simulink model "ur5_simulink_ros2_pbvs_all_methods_2023b"  (R2023b)
settings: Solver=ode4  StartTime=0.0  StopTime=inf  FixedStep=0.005  RelTol=1e-3
InitFcn:
  | l=5;
model workspace (MAT data in the model file):
  SL_ROS_VariableLengthArrays_MaxSizes.CommonInfo.ArrayTruncateAction = 'EmitWarning'
  SL_ROS_VariableLengthArrays_MaxSizes.MsgTypeMap = containers.Map
  SL_ROS_VariableLengthArrays_MaxSizes.MsgTypeMap.serialization.keys = {'example_interfaces/Float64MultiArray'}
  SL_ROS_VariableLengthArrays_MaxSizes.MsgTypeMap.serialization.values{1}.PropertyName = 'data'
  SL_ROS_VariableLengthArrays_MaxSizes.MsgTypeMap.serialization.values{1}.DataType = 'double'
  SL_ROS_VariableLengthArrays_MaxSizes.MsgTypeMap.serialization.values{1}.MaxLength = 1
  SL_ROS_VariableLengthArrays_MaxSizes.MsgTypeMap.serialization.uniformity = 0
  SL_ROS_VariableLengthArrays_MaxSizes.MsgTypeMap.serialization.keyType = 'char'
  SL_ROS_VariableLengthArrays_MaxSizes.MsgTypeMap.serialization.valueType = 'any'
values from neighbouring files (symbols this model uses):
  D = zeros(6,12)    [ibvs_cstate.m]
undefined symbols (not defined in the file or in its folder): data, data_SL_Info, DiscIntNeverNeededParam
libraries: simulink x9, ros2lib x8, slpidlib x6, robotmaniplib x3, mpclib x3, robotcorelib x1
(part 1 of 2)
settings Model: SimulationMode=accelerator  Creator=81232  LastModifiedBy=Administrator
settings OptimizationCC: EnhancedBackFolding=on  PassReuseOutputArgsAs=Individual arguments  ZeroExternalMemoryAtStartup=off  ZeroInternalMemoryAtStartup=off  MaxStackSize=64  OptimizeBlockOrder=speed  DifferentSizesBufferReuse=on  OptimizationCustomize=off  EfficientTunableParamExpr=on
settings DebuggingCC: ParameterTunabilityLossMsg=error
settings ModelReferenceCC: EnableRefExpFcnMdlSchedulingChecks=on
settings SFSimCC: MATLABDynamicMemAlloc=off
settings RTWCC: Description=Embedded Coder  SystemTargetFile=ert.tlc  HardwareBoard=Robot Operating System 2 (ROS 2)  TLCOptions="-aInlineSetEventsForThisBaseRateFcn=TLC_FALSE -aSuppressMultiTaskScheduler=TLC_FALSE  -aRateBasedStepFcn=0"  TemplateMakefile=ert_default_tmf  Toolchain=Colcon Tools  TargetLang=C++
settings CodeAppCC: ForceParamTrailComments=on  IgnoreCustomStorageClasses=off  OperatorAnnotations=on  SimulinkDataObjDesc=on  SFDataObjDesc=on  InsertBlockDesc=on
settings ERTTargetCC: CodeInterfacePackaging=C++ class  RootIOFormat=Structure reference

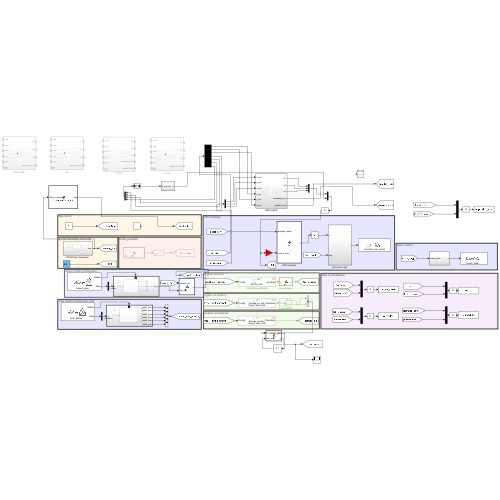
[thumbnail: Simulink's stored preview of the top-level diagram]
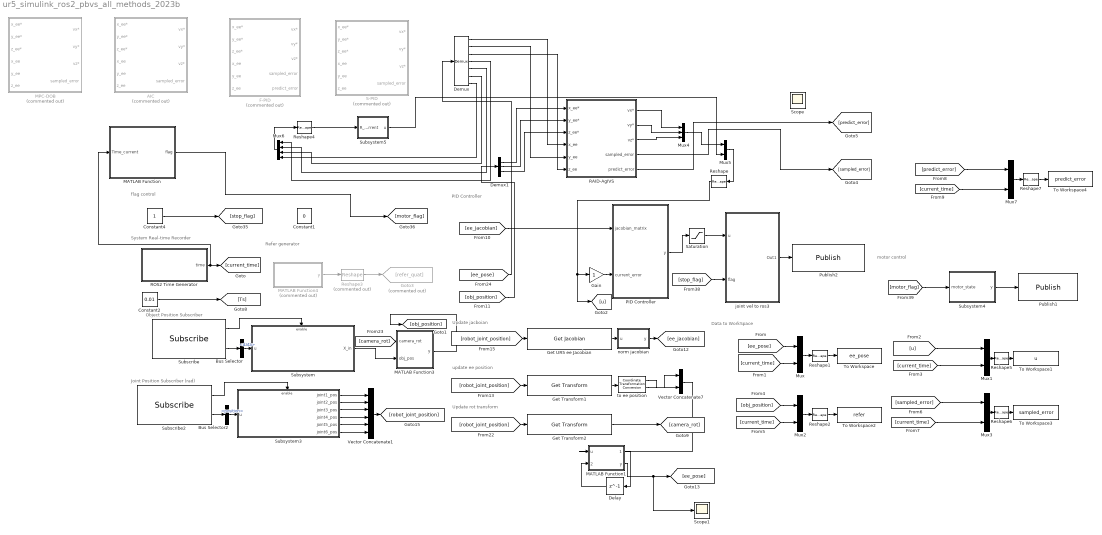
== system ur5_simulink_ros2_pbvs_all_methods_2023b ==
  note: PID Controller
  note: update ee position
  note: Joint Position Subscriber (rad)
  note: Refer generator
  note: Data to WorkSpace
  note: System Real-time Recorder
  note: Object Position Subscriber
  note: Update jacboian
  note: Update rot transform
  note: flag control
  note: motor control
  AIC : Subsystem  Commented=on
  Bus Selector : BusSelector  OutputSignals=data
  Bus Selector2 : BusSelector  OutputSignals=position
  Constant1 : Constant  Value=0
  Constant2 : Constant  Value=0.01
  Constant4 : Constant
  Delay : Delay  DelayLength=1  InitialCondition=[0;0;0;0]
  Demux : Demux  Outputs=7
  Demux1 : Demux  Outputs=3
  F-PID : Subsystem  Commented=on
  Gain : Gain
  Get Transform1 : robotmaniplib/Get Transform  RigidBodyTree=ur5_model  SourceBody=ee_link  TargetBody=base_link  SimulateUsing=Interpreted execution
  Get Transform2 : robotmaniplib/Get Transform  RigidBodyTree=ur5_model  SourceBody=camera  TargetBody=base_link  SimulateUsing=Interpreted execution
  Get UR5 ee Jacobian : robotmaniplib/Get Jacobian  RigidBodyTree=ur5_model  EndEffector=ee_link  SimulateUsing=Interpreted execution
  Goto3 : Goto  Commented=on  GotoTag=refer_quat
  MATLAB Function : MATLAB Function  TreatAsAtomicUnit=on
  MATLAB Function1 : MATLAB Function  TreatAsAtomicUnit=on
  MATLAB Function3 : MATLAB Function  TreatAsAtomicUnit=on
  MATLAB Function4 : MATLAB Function  Commented=on  TreatAsAtomicUnit=on
  MPC-DOB : Subsystem  Commented=on
  Mux{,1..3,5,7} (6 alike) : Mux  Inputs=2
  Mux4 : Mux  Inputs=3
  Mux6 : Mux
  PID Controller : MATLAB Function  TreatAsAtomicUnit=on
  Publish1 : ros2lib/Publish  topicSource=Select from ROS network  topic=/motor_state  messageType=std_msgs/Int64  QOSHistory=Keep last  QOSDepth=1  QOSReliability=Reliable  QOSDurability=Volatile
      settings: LibrarySourceBlock=roslib/ROS 2/Publish
  Publish2 : ros2lib/Publish  topicSource=Select from ROS network  topic=/simulink_mpc_result  messageType=std_msgs/Float64MultiArray  QOSHistory=Keep last  QOSDepth=1  QOSReliability=Reliable  QOSDurability=Volatile
      settings: LibrarySourceBlock=roslib/ROS 2/Publish
  RAID-AgIVS : Subsystem
  ROS2 Time Generator : Subsystem
  Reshape : Reshape  OutputDimensionality=Customize  OutputDimensions=[6,1]
  Reshape1 : Reshape  OutputDimensionality=Customize  OutputDimensions=[8]
  Reshape2 : Reshape  OutputDimensionality=Customize  OutputDimensions=[4]
  Reshape3 : Reshape  Commented=on  OutputDimensions=[1,7]
  Reshape4 : Reshape  OutputDimensionality=Row vector (2-D)
  Reshape5 : Reshape  OutputDimensionality=Customize  OutputDimensions=[7]
  Reshape6 : Reshape  OutputDimensionality=Customize  OutputDimensions=[4]
  Reshape7 : Reshape  OutputDimensionality=Customize  OutputDimensions=[4]
  S-PID : Subsystem  Commented=on
  Saturation : Saturate  UpperLimit=0.7  LowerLimit=-0.7  LinearizeAsGain=off
  Scope : Scope
  Scope1 : Scope
  Subscribe : ros2lib/Subscribe  topicSource=Select from ROS network  topic=/object_pose  messageType=std_msgs/Float64MultiArray  sampleTime=-1  QOSHistory=Keep last  QOSDepth=1  QOSReliability=Reliable  QOSDurability=Volatile
  Subscribe2 : ros2lib/Subscribe  topicSource=Select from ROS network  topic=/joint_states  messageType=sensor_msgs/JointState  sampleTime=-1  QOSHistory=Keep last  QOSDepth=1  QOSReliability=Reliable  QOSDurability=Volatile
  Subsystem : Subsystem
  Subsystem3 : Subsystem
  Subsystem4 : Subsystem
  Subsystem5 : Subsystem
  To Workspace : ToWorkspace  VariableName=ee_pose  SaveFormat=Timeseries  SampleTime=-1
  To Workspace1 : ToWorkspace  VariableName=u  SaveFormat=Timeseries  SampleTime=-1
  To Workspace2 : ToWorkspace  VariableName=refer  SaveFormat=Timeseries  SampleTime=-1
  To Workspace3 : ToWorkspace  VariableName=sampled_error  SaveFormat=Timeseries  SampleTime=-1
  To Workspace4 : ToWorkspace  VariableName=predict_error  SaveFormat=Timeseries  SampleTime=-1
  Vector Concatenate1 : Concatenate  NumInputs=6
  Vector Concatenate7 : Concatenate
  joint vel to ros3 : Subsystem
  norm jacobian : MATLAB Function  TreatAsAtomicUnit=on
  to ee position : robotcorelib/Coordinate Transformation Conversion  InputRepresentation=Homogeneous Transformation  InputEulerSequence=ZYX  ShowTrVecInputPort=on  OutputRepresentation=Quaternion  OutputEulerSequence=ZYX  ShowTrVecOutputPort=on  SimulateUsing=Interpreted execution
  wires:
  Bus Selector/1 -> Subsystem/1(u)  "<data>"
  Subscribe/2 -> Bus Selector/1
  Subscribe/1 -> Subsystem/Enable
  ROS2 Time Generator/1(time) -> [current_time], MATLAB Function/1(Time_current)
  [ee_pose] -> Mux/1
  [current_time] -> Mux/2
  [current_time] -> Mux1/2
  [current_time] -> Mux2/2
  Mux2/1 -> Reshape2/1
  [current_time] -> Mux3/2
  Mux3/1 -> Reshape6/1
  [sampled_error] -> Mux3/1
  [u] -> Mux1/1
  Mux1/1 -> Reshape5/1
  Reshape5/1 -> To Workspace1/1
  Reshape6/1 -> To Workspace3/1
  Subscribe2/2 -> Bus Selector2/1
  Bus Selector2/1 -> Subsystem3/1(u)  "<position>"
  Subscribe2/1 -> Subsystem3/Enable
  Subsystem3/1(joint1_pos) -> Vector Concatenate1/1
  Subsystem3/2(joint2_pos) -> Vector Concatenate1/2
  Subsystem3/3(joint3_pos) -> Vector Concatenate1/3
  Subsystem3/4(joint4_pos) -> Vector Concatenate1/4
  Subsystem3/5(joint5_pos) -> Vector Concatenate1/5
  Subsystem3/6(joint6_pos) -> Vector Concatenate1/6
  norm jacobian/1(y) -> [ee_jacobian]
  Get UR5 ee Jacobian/1 -> norm jacobian/1(u)
  [robot_joint_position] -> Get UR5 ee Jacobian/1
  [robot_joint_position] -> Get Transform1/1
  Vector Concatenate1/1 -> [robot_joint_position]
  Mux/1 -> Reshape1/1
  Reshape1/1 -> To Workspace/1
  Reshape2/1 -> To Workspace2/1
  [obj_position] -> Mux2/1
  Constant2/1 -> [Ts]
  Get Transform2/1 -> [camera_rot]
  MATLAB Function3/1(y) -> [obj_position]
  [camera_rot] -> MATLAB Function3/1(camera_rot)
  Subsystem/1(X_in) -> MATLAB Function3/2(obj_pos)
  Reshape3/1 -> Goto3/1
  MATLAB Function4/1(y) -> Reshape3/1
  Get Transform1/1 -> to ee position/1
  to ee position/1 -> Vector Concatenate7/2
  to ee position/2 -> Vector Concatenate7/1
  [ee_jacobian] -> PID Controller/1(jacobian_matrix)
  Saturation/1 -> joint vel to ros3/1(u)
  joint vel to ros3/1(Out1) -> Publish2/1
  PID Controller/1(y) -> Saturation/1
  Constant4/1 -> [stop_flag]
  [stop_flag] -> joint vel to ros3/2(flag)
  Mux5/1 -> Reshape/1
  Gain/1 -> PID Controller/2(current_error)
  Subsystem4/1(y) -> Publish1/1
  [motor_flag] -> Subsystem4/1(motor_state)
  [robot_joint_position] -> Get Transform2/1
  Demux/1 -> RAID-AgIVS/4(x_ee)
  Demux/2 -> RAID-AgIVS/5(y_ee)
  Demux/3 -> RAID-AgIVS/6(z_ee)
  Demux1/1 -> RAID-AgIVS/1(x_ee*)
  Demux1/2 -> RAID-AgIVS/2(y_ee*)
  Demux1/3 -> RAID-AgIVS/3(z_ee*)
  Mux4/1 -> Mux5/1
  Reshape/1 -> [u], Gain/1
  [ee_pose] -> Demux/1
  [obj_position] -> Demux1/1
  RAID-AgIVS/1(vx*) -> Mux4/1
  Demux/4 -> Mux6/1
  Demux/5 -> Mux6/2
  Demux/6 -> Mux6/3
  Demux/7 -> Mux6/4
  Mux6/1 -> Reshape4/1
  Subsystem5/1(u) -> Mux5/2
  Reshape4/1 -> Subsystem5/1(R_current)
  [current_time] -> Mux7/2
  [predict_error] -> Mux7/1
  Mux7/1 -> Reshape7/1
  Reshape7/1 -> To Workspace4/1
  Vector Concatenate7/1 -> MATLAB Function1/1(u)
  MATLAB Function1/1(current_quat) -> Delay/1
  Delay/1 -> MATLAB Function1/2(last_quat)
  MATLAB Function1/2(y) -> Scope1/1, [ee_pose]
  RAID-AgIVS/2(vy*) -> Mux4/2
  MATLAB Function/1(flag) -> [motor_flag]
  RAID-AgIVS/5(predict_error) -> [predict_error]
  RAID-AgIVS/3(vz*) -> Mux4/3
  RAID-AgIVS/4(sampled_error) -> [sampled_error]

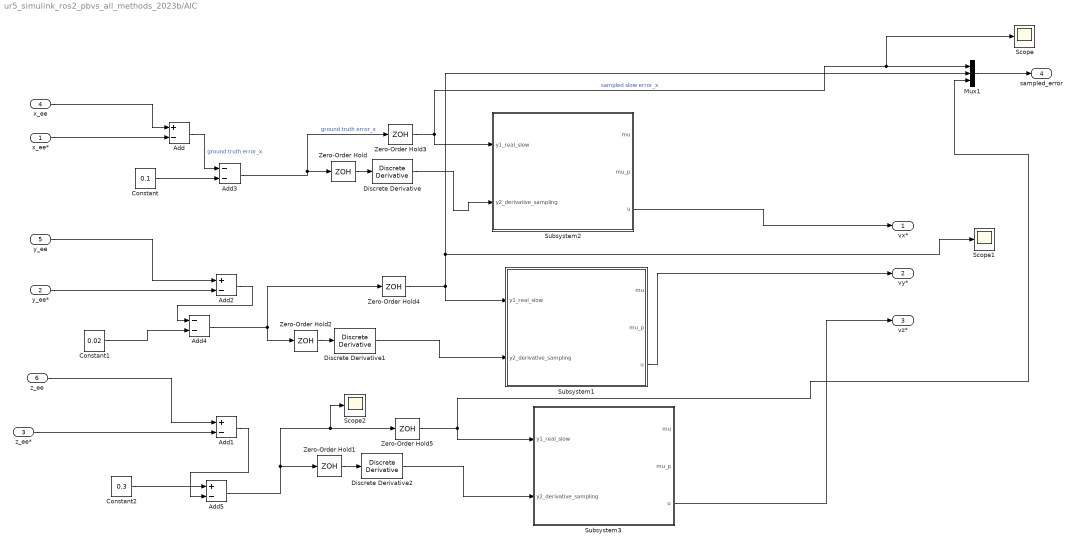
== system ur5_simulink_ros2_pbvs_all_methods_2023b/AIC ==
  x_ee* : Inport
  y_ee* : Inport  Port=2
  z_ee* : Inport  Port=3
  x_ee : Inport  Port=4
  y_ee : Inport  Port=5
  z_ee : Inport  Port=6
  Add{,1..2,5} (4 alike) : Sum  Inputs=+-
  Add3 : Sum  Inputs=--
  Add4 : Sum  Inputs=--
  Constant : Constant  Value=0.1
  Constant1 : Constant  Value=0.02
  Constant2 : Constant  Value=0.3
  Discrete Derivative : simulink/Discrete/Discrete Derivative  gainval=1.0  ICPrevScaledInput=0  OutMin=[]  OutMax=[]  OutDataType=fixdt(1, 16)  OutScaling=2^-10  DoSatur=off
  Discrete Derivative1 : simulink/Discrete/Discrete Derivative  gainval=1.0  ICPrevScaledInput=0.0  OutMin=[]  OutMax=[]  OutDataType=fixdt(1, 16)  OutScaling=2^-10  DoSatur=off
  Discrete Derivative2 : simulink/Discrete/Discrete Derivative  gainval=1.0  ICPrevScaledInput=0.0  OutMin=[]  OutMax=[]  OutDataType=fixdt(1, 16)  OutScaling=2^-10  DoSatur=off
  Mux1 : Mux  Inputs=3
  Scope : Scope
  Scope1 : Scope
  Scope2 : Scope
  Subsystem1 : Subsystem
  Subsystem2 : Subsystem
  Subsystem3 : Subsystem
  Zero-Order Hold{,1..5} (6 alike) : ZeroOrderHold  SampleTime=0.05
  vx* : Outport
  vy* : Outport  Port=2
  vz* : Outport  Port=3
  sampled_error : Outport  Port=4
  wires:
  Subsystem3/3(u) -> vz*/1
  Subsystem1/3(u) -> vy*/1
  Subsystem2/3(u) -> vx*/1
  Discrete Derivative1/1 -> Subsystem1/2(y2_derivative_sampling)
  Add1/1 -> Add5/2
  Constant/1 -> Add3/2
  Add/1 -> Add3/1  "ground truth error_x"
  z_ee*/1 -> Add1/2
  Discrete Derivative/1 -> Subsystem2/2(y2_derivative_sampling)
  y_ee*/1 -> Add2/2
  Constant2/1 -> Add5/1
  Zero-Order Hold5/1 -> Subsystem3/1(y1_real_slow), Mux1/3
  Add4/1 -> Zero-Order Hold4/1, Zero-Order Hold2/1
  x_ee*/1 -> Add/2
  x_ee/1 -> Add/1
  Zero-Order Hold1/1 -> Discrete Derivative2/1
  Zero-Order Hold/1 -> Discrete Derivative/1
  Add5/1 -> Zero-Order Hold5/1, Scope2/1, Zero-Order Hold1/1
  Zero-Order Hold3/1 -> Scope/1, Mux1/1, Subsystem2/1(y1_real_slow)  "sampled slow error_x"
  Zero-Order Hold2/1 -> Discrete Derivative1/1
  y_ee/1 -> Add2/1
  Add2/1 -> Add4/1
  Constant1/1 -> Add4/2
  Zero-Order Hold4/1 -> Subsystem1/1(y1_real_slow), Scope1/1, Mux1/2
  z_ee/1 -> Add1/1
  Add3/1 -> Zero-Order Hold3/1, Zero-Order Hold/1  "ground truth error_x"
  Discrete Derivative2/1 -> Subsystem3/2(y2_derivative_sampling)
  Mux1/1 -> sampled_error/1

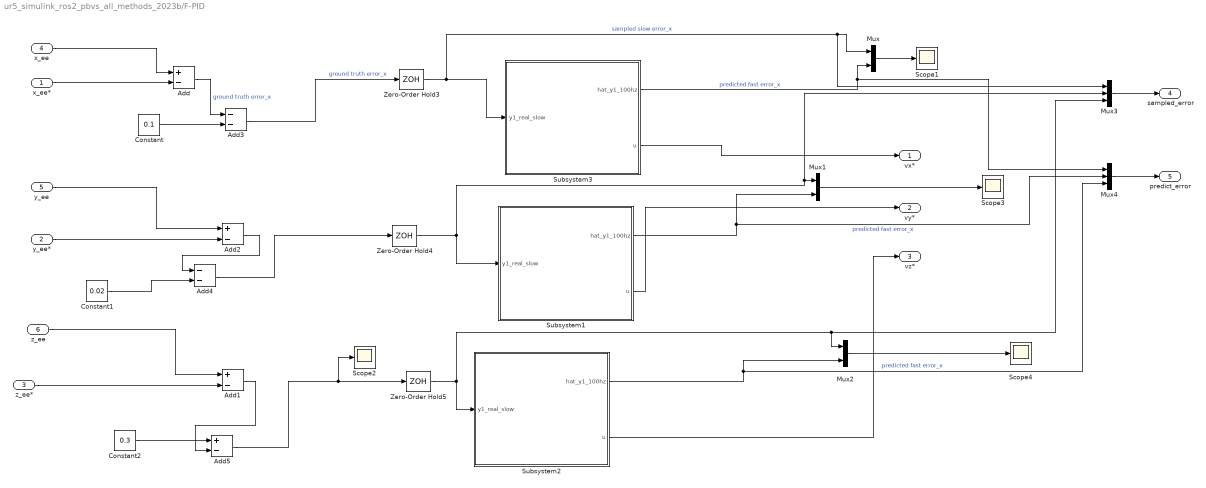
== system ur5_simulink_ros2_pbvs_all_methods_2023b/F-PID ==
  x_ee* : Inport
  y_ee* : Inport  Port=2
  z_ee* : Inport  Port=3
  x_ee : Inport  Port=4
  y_ee : Inport  Port=5
  z_ee : Inport  Port=6
  Add{,1..2,5} (4 alike) : Sum  Inputs=+-
  Add3 : Sum  Inputs=--
  Add4 : Sum  Inputs=--
  Constant : Constant  Value=0.1
  Constant1 : Constant  Value=0.02
  Constant2 : Constant  Value=0.3
  Mux : Mux  Inputs=2
  Mux1 : Mux  Inputs=2
  Mux2 : Mux  Inputs=2
  Mux3 : Mux  Inputs=3
  Mux4 : Mux  Inputs=3
  Scope{1..4} (4 alike) : Scope
  Subsystem1 : Subsystem
  Subsystem2 : Subsystem
  Subsystem3 : Subsystem
  Zero-Order Hold3 : ZeroOrderHold  SampleTime=0.05
  Zero-Order Hold4 : ZeroOrderHold  SampleTime=0.05
  Zero-Order Hold5 : ZeroOrderHold  SampleTime=0.05
  vx* : Outport
  vy* : Outport  Port=2
  vz* : Outport  Port=3
  sampled_error : Outport  Port=4
  predict_error : Outport  Port=5
  wires:
  Add4/1 -> Zero-Order Hold4/1
  x_ee/1 -> Add/1
  Add5/1 -> Zero-Order Hold5/1, Scope2/1
  Subsystem3/2(u) -> vx*/1
  Add3/1 -> Zero-Order Hold3/1  "ground truth error_x"
  x_ee*/1 -> Add/2
  y_ee/1 -> Add2/1
  z_ee/1 -> Add1/1
  Subsystem2/2(u) -> vz*/1
  y_ee*/1 -> Add2/2
  z_ee*/1 -> Add1/2
  Zero-Order Hold3/1 -> Mux3/1, Mux/1, Subsystem3/1(y1_real_slow)  "sampled slow error_x"
  Zero-Order Hold4/1 -> Subsystem1/1(y1_real_slow), Mux3/2, Mux1/1
  Subsystem1/2(u) -> vy*/1
  Subsystem3/1(hat_y1_100hz) -> Mux4/1, Mux/2  "predicted fast error_x"
  Mux/1 -> Scope1/1
  Add/1 -> Add3/1  "ground truth error_x"
  Constant/1 -> Add3/2
  Constant1/1 -> Add4/2
  Add2/1 -> Add4/1
  Constant2/1 -> Add5/1
  Add1/1 -> Add5/2
  Subsystem1/1(hat_y1_100hz) -> Mux4/2, Mux1/2  "predicted fast error_x"
  Mux1/1 -> Scope3/1
  Mux2/1 -> Scope4/1
  Zero-Order Hold5/1 -> Subsystem2/1(y1_real_slow), Mux3/3, Mux2/1
  Subsystem2/1(hat_y1_100hz) -> Mux4/3, Mux2/2  "predicted fast error_x"
  Mux3/1 -> sampled_error/1
  Mux4/1 -> predict_error/1

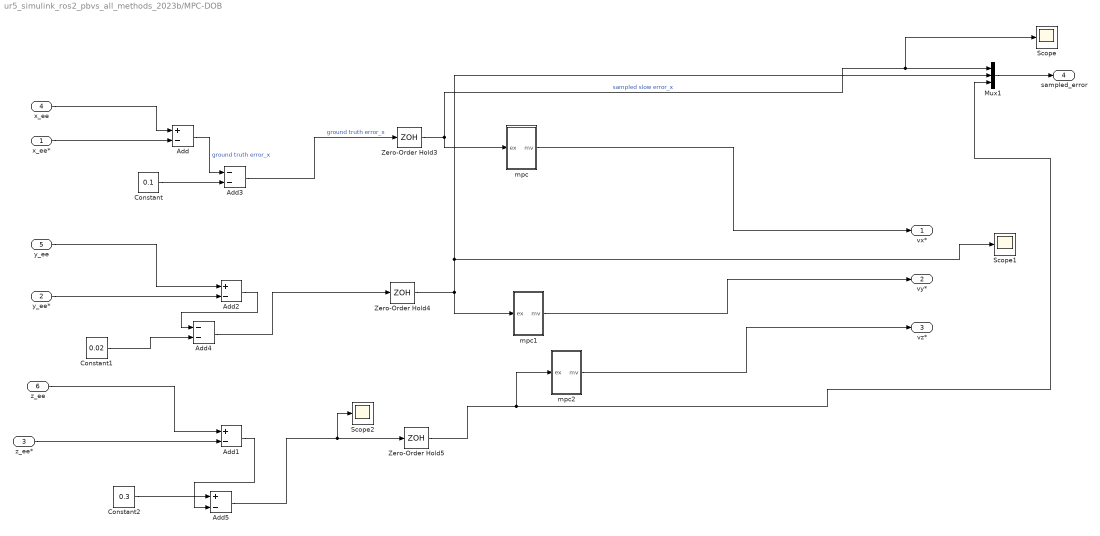
== system ur5_simulink_ros2_pbvs_all_methods_2023b/MPC-DOB ==
  x_ee* : Inport
  y_ee* : Inport  Port=2
  z_ee* : Inport  Port=3
  x_ee : Inport  Port=4
  y_ee : Inport  Port=5
  z_ee : Inport  Port=6
  Add{,1..2,5} (4 alike) : Sum  Inputs=+-
  Add3 : Sum  Inputs=--
  Add4 : Sum  Inputs=--
  Constant : Constant  Value=0.1
  Constant1 : Constant  Value=0.02
  Constant2 : Constant  Value=0.3
  Mux1 : Mux  Inputs=3
  Scope : Scope
  Scope1 : Scope
  Scope2 : Scope
  Zero-Order Hold3 : ZeroOrderHold  SampleTime=0.05
  Zero-Order Hold4 : ZeroOrderHold  SampleTime=0.05
  Zero-Order Hold5 : ZeroOrderHold  SampleTime=0.05
  mpc : Subsystem
  mpc1 : Subsystem
  mpc2 : Subsystem
  vx* : Outport
  vy* : Outport  Port=2
  vz* : Outport  Port=3
  sampled_error : Outport  Port=4
  wires:
  mpc2/1(mv) -> vz*/1
  mpc1/1(mv) -> vy*/1
  mpc/1(mv) -> vx*/1
  Add1/1 -> Add5/2
  Constant/1 -> Add3/2
  Add/1 -> Add3/1  "ground truth error_x"
  z_ee*/1 -> Add1/2
  y_ee*/1 -> Add2/2
  Constant2/1 -> Add5/1
  Zero-Order Hold5/1 -> mpc2/1(ex), Mux1/3
  Add4/1 -> Zero-Order Hold4/1
  x_ee*/1 -> Add/2
  x_ee/1 -> Add/1
  Add5/1 -> Zero-Order Hold5/1, Scope2/1
  Zero-Order Hold3/1 -> mpc/1(ex), Scope/1, Mux1/1  "sampled slow error_x"
  y_ee/1 -> Add2/1
  Add2/1 -> Add4/1
  Constant1/1 -> Add4/2
  Zero-Order Hold4/1 -> mpc1/1(ex), Scope1/1, Mux1/2
  z_ee/1 -> Add1/1
  Add3/1 -> Zero-Order Hold3/1  "ground truth error_x"
  Mux1/1 -> sampled_error/1

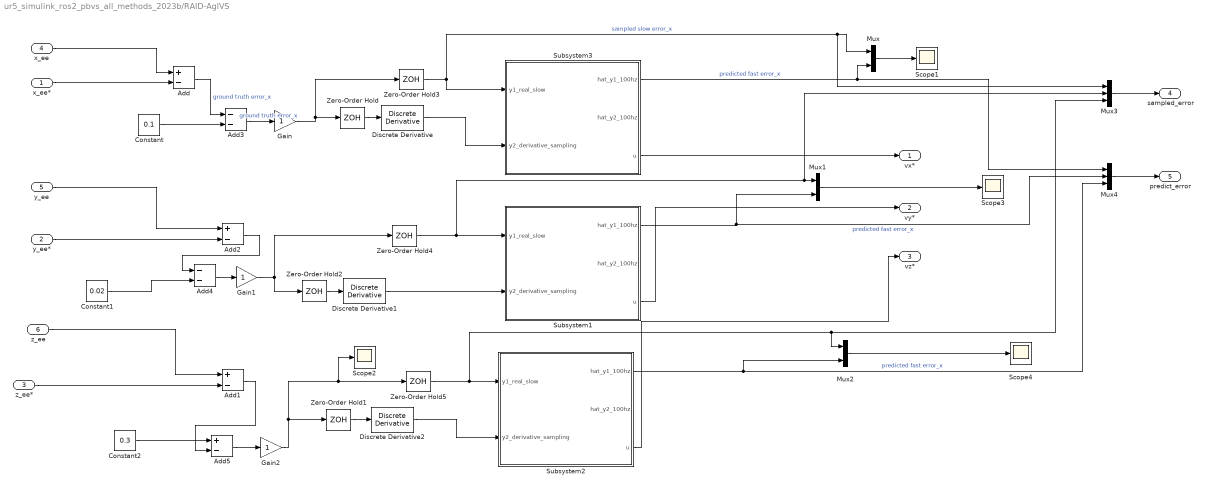
== system ur5_simulink_ros2_pbvs_all_methods_2023b/RAID-AgIVS ==
  x_ee* : Inport
  y_ee* : Inport  Port=2
  z_ee* : Inport  Port=3
  x_ee : Inport  Port=4
  y_ee : Inport  Port=5
  z_ee : Inport  Port=6
  Add{,1..2,5} (4 alike) : Sum  Inputs=+-
  Add3 : Sum  Inputs=--
  Add4 : Sum  Inputs=--
  Constant : Constant  Value=0.1
  Constant1 : Constant  Value=0.02
  Constant2 : Constant  Value=0.3
  Discrete Derivative : simulink/Discrete/Discrete Derivative  gainval=1.0  ICPrevScaledInput=0  OutMin=[]  OutMax=[]  OutDataType=fixdt(1, 16)  OutScaling=2^-10  DoSatur=off
  Discrete Derivative1 : simulink/Discrete/Discrete Derivative  gainval=1.0  ICPrevScaledInput=0.0  OutMin=[]  OutMax=[]  OutDataType=fixdt(1, 16)  OutScaling=2^-10  DoSatur=off
  Discrete Derivative2 : simulink/Discrete/Discrete Derivative  gainval=1.0  ICPrevScaledInput=0.0  OutMin=[]  OutMax=[]  OutDataType=fixdt(1, 16)  OutScaling=2^-10  DoSatur=off
  Gain : Gain
  Gain1 : Gain
  Gain2 : Gain
  Mux : Mux  Inputs=2
  Mux1 : Mux  Inputs=2
  Mux2 : Mux  Inputs=2
  Mux3 : Mux  Inputs=3
  Mux4 : Mux  Inputs=3
  Scope{1..4} (4 alike) : Scope
  Subsystem1 : Subsystem
  Subsystem2 : Subsystem
  Subsystem3 : Subsystem
  Zero-Order Hold{,1..5} (6 alike) : ZeroOrderHold  SampleTime=0.05
  vx* : Outport
  vy* : Outport  Port=2
  vz* : Outport  Port=3
  sampled_error : Outport  Port=4
  predict_error : Outport  Port=5
  wires:
  Add4/1 -> Gain1/1
  x_ee/1 -> Add/1
  Discrete Derivative/1 -> Subsystem3/2(y2_derivative_sampling)
  Zero-Order Hold/1 -> Discrete Derivative/1
  Discrete Derivative1/1 -> Subsystem1/2(y2_derivative_sampling)
  Add5/1 -> Gain2/1
  Subsystem3/3(u) -> vx*/1
  Add3/1 -> Gain/1  "ground truth error_x"
  x_ee*/1 -> Add/2
  y_ee/1 -> Add2/1
  z_ee/1 -> Add1/1
  Subsystem2/3(u) -> vz*/1
  Zero-Order Hold1/1 -> Discrete Derivative2/1
  Zero-Order Hold2/1 -> Discrete Derivative1/1
  y_ee*/1 -> Add2/2
  z_ee*/1 -> Add1/2
  Zero-Order Hold3/1 -> Mux3/1, Mux/1, Subsystem3/1(y1_real_slow)  "sampled slow error_x"
  Zero-Order Hold4/1 -> Mux3/2, Mux1/1, Subsystem1/1(y1_real_slow)
  Subsystem1/3(u) -> vy*/1
  Subsystem3/1(hat_y1_100hz) -> Mux4/1, Mux/2  "predicted fast error_x"
  Mux/1 -> Scope1/1
  Discrete Derivative2/1 -> Subsystem2/2(y2_derivative_sampling)
  Add/1 -> Add3/1  "ground truth error_x"
  Constant/1 -> Add3/2
  Constant1/1 -> Add4/2
  Add2/1 -> Add4/1
  Constant2/1 -> Add5/1
  Add1/1 -> Add5/2
  Subsystem1/1(hat_y1_100hz) -> Mux4/2, Mux1/2  "predicted fast error_x"
  Mux1/1 -> Scope3/1
  Mux2/1 -> Scope4/1
  Zero-Order Hold5/1 -> Mux3/3, Mux2/1, Subsystem2/1(y1_real_slow)
  Subsystem2/1(hat_y1_100hz) -> Mux4/3, Mux2/2  "predicted fast error_x"
  Mux3/1 -> sampled_error/1
  Mux4/1 -> predict_error/1
  Gain/1 -> Zero-Order Hold3/1, Zero-Order Hold/1
  Gain1/1 -> Zero-Order Hold4/1, Zero-Order Hold2/1
  Gain2/1 -> Zero-Order Hold5/1, Scope2/1, Zero-Order Hold1/1

== system ur5_simulink_ros2_pbvs_all_methods_2023b/ROS2 Time Generator ==
  Current Time : ros2lib/Current Time  OutputFormat=double  SampleTime=-1  ModelName=ur5_simulink_ros2_pbvs_all_methods_2023b
      settings: LibrarySourceBlock=roslib/ROS 2/Current Time
  Current Time1 : ros2lib/Current Time  OutputFormat=double  SampleTime=-1  ModelName=ur5_simulink_ros2_pbvs_all_methods_2023b
      settings: LibrarySourceBlock=roslib/ROS 2/Current Time
  Delay : Delay  DelayLength=1  InitialConditionSource=Input port
      settings: InputPortMap=u0,p4
  MATLAB Function : MATLAB Function  TreatAsAtomicUnit=on
  time : Outport
  wires:
  Delay/1 -> MATLAB Function/2(last_time)
  Current Time1/1 -> Delay/2
  MATLAB Function/2(init_time) -> Delay/1
  Current Time/1 -> MATLAB Function/1(current_time)
  MATLAB Function/1(time_x) -> time/1

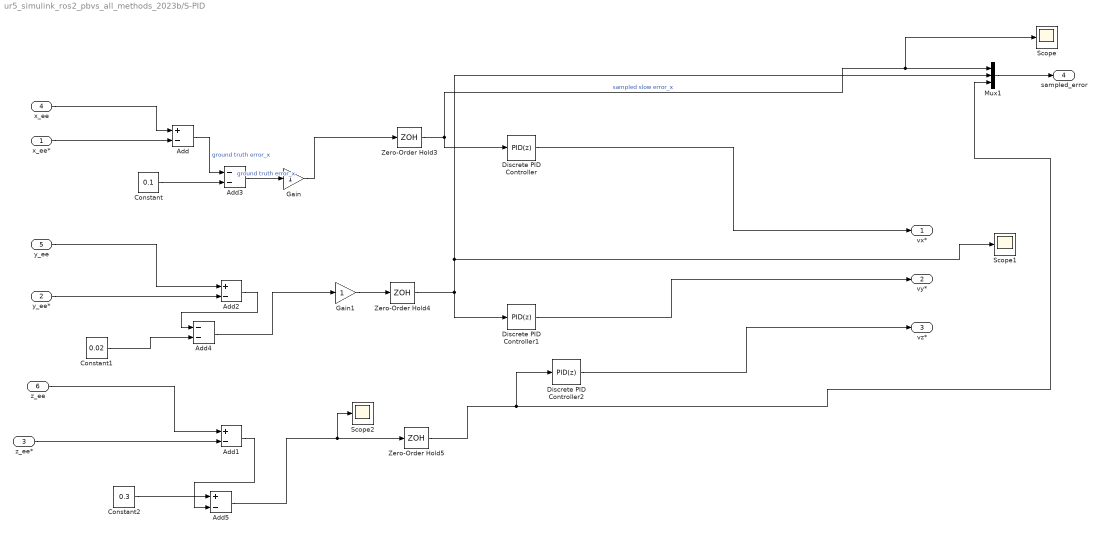
== system ur5_simulink_ros2_pbvs_all_methods_2023b/S-PID ==
  x_ee* : Inport
  y_ee* : Inport  Port=2
  z_ee* : Inport  Port=3
  x_ee : Inport  Port=4
  y_ee : Inport  Port=5
  z_ee : Inport  Port=6
  Add{,1..2,5} (4 alike) : Sum  Inputs=+-
  Add3 : Sum  Inputs=--
  Add4 : Sum  Inputs=--
  Constant : Constant  Value=0.1
  Constant1 : Constant  Value=0.02
  Constant2 : Constant  Value=0.3
  Discrete PID Controller : slpidlib/PID Controller  Controller=PID  Form=Parallel  TimeDomain=Discrete-time  UseExternalTs=off  SampleTime=0.05  IntegratorMethod=Forward Euler  FilterMethod=Forward Euler  ControllerParametersSource=internal  P=4.5  I=4.3  UseKiTs=off  D=0  N=100  UseFilter=on  TunerSelectOption=Transfer Function Based (PID Tuner App)  InitialConditionSource=internal  InitialConditionForIntegrator=0  InitialConditionForFilter=0  DifferentiatorICPrevScaledInput=0  ExternalReset=none  TrackingMode=off  Kt=1  LimitOutput=off  SatLimitsSource=internal  UpperSaturationLimit=inf  LowerSaturationLimit=-inf  LinearizeAsGain=off  AntiWindupMode=none  Kb=1  LimitIntegrator=off  UpperIntegratorSaturationLimit=inf  LowerIntegratorSaturationLimit=-inf  POutMin=[]  POutMax=[]  IOutMin=[]  IOutMax=[]  DOutMin=[]  DOutMax=[]  NOutMin=[]  NOutMax=[]  SumOutMin=[]  SumOutMax=[]  SaturationOutMin=[]  SaturationOutMax=[]  PParamMin=[]  PParamMax=[]  IParamMin=[]  IParamMax=[]  DParamMin=[]  DParamMax=[]  NParamMin=[]  NParamMax=[]  KbParamMin=[]  KbParamMax=[]  KtParamMin=[]  KtParamMax=[]  KbOutMin=[]  KbOutMax=[]  KtOutMin=[]  KtOutMax=[]  IntegratorOutMin=[]  IntegratorOutMax=[]  FilterOutMin=[]  FilterOutMax=[]  SumI1OutMin=[]  SumI1OutMax=[]  SumI2OutMin=[]  SumI2OutMax=[]  SumI3OutMin=[]  SumI3OutMax=[]  SumI4OutMin=[]  SumI4OutMax=[]  SumDOutMin=[]  SumDOutMax=[]  DifferentiatorOutMin=[]  DifferentiatorOutMax=[]  FilterDiffOutCoefMin=[]  FilterDiffOutCoefMax=[]  ReciprocalOutMin=[]  ReciprocalOutMax=[]  SumDenOutMin=[]  SumDenOutMax=[]  SumNumOutMin=[]  SumNumOutMax=[]  DivideOutMin=[]  DivideOutMax=[]  UdiffTsProdOutMin=[]  UdiffTsProdOutMax=[]  NTsProdOutMin=[]  NTsProdOutMax=[]  UintegralTsProdOutMin=[]  UintegralTsProdOutMax=[]  UngainTsProdOutMin=[]  UngainTsProdOutMax=[]  ClampingZeroOutDataTypeStr=Inherit: Inherit via back propagation  ClampingZeroOutMin=[]  ClampingZeroOutMax=[]  FilterDenConstantOutDataTypeStr=Inherit: Inherit via back propagation  FilterDenConstantOutMin=[]  FilterDenConstantOutMax=[]  PCopyOutDataTypeStr=Inherit: Inherit via back propagation  PCopyOutMin=[]  PCopyOutMax=[]  NCopyOutDataTypeStr=Inherit: Inherit via back propagation  NCopyOutMin=[]  NCopyOutMax=[]  IntegratorContinuousStateAttributes=''  IntegratorStateMustResolveToSignalObject=off  IntegratorRTWStateStorageClass=Auto  FilterContinuousStateAttributes=''  FilterStateMustResolveToSignalObject=off  FilterRTWStateStorageClass=Auto  ParallelPVariant=InternalParameters  IdealPVariant=Disabled  IVariant=InternalParameters  DVariant=InternalParameters  IntegratorVariant=Discrete  SatVariant=Disabled  AWVariant=Passthrough  PCopyVariant=Disabled  TRVariant=Disabled  FdbkBlocksVariant=Forward  IdealPFdbkVariant=Disabled  SatFdbkVariant=Disabled  DerivativeFilterVariant=ForwardEulerFilter  NVariant=InternalParameters  NCopyVariant=Disabled  FilterICVariant=InternalICsFilter  IntegratorICVariant=InternalICs  ExternalResetVariant=Disabled  TRSumVariant=Passthrough  SumFdbkVariant=Disabled  SumVariant=Sum_PID  TsampFilterVariant=InternalTs  TsampNgainVariant=Passthrough  TsampIntegralVariant=Disabled_SignalSpec  ExternalSaturationOutDataTypeStr=Inherit: Same as second input
      settings: LibrarySourceBlock=simulink/Discrete/Discrete PID Controller
  Discrete PID Controller1 : slpidlib/PID Controller  Controller=PID  Form=Parallel  TimeDomain=Discrete-time  UseExternalTs=off  SampleTime=0.05  IntegratorMethod=Forward Euler  FilterMethod=Forward Euler  ControllerParametersSource=internal  P=4.5  I=4.3  UseKiTs=off  D=0  N=100  UseFilter=on  TunerSelectOption=Transfer Function Based (PID Tuner App)  InitialConditionSource=internal  InitialConditionForIntegrator=0  InitialConditionForFilter=0  DifferentiatorICPrevScaledInput=0  ExternalReset=none  TrackingMode=off  Kt=1  LimitOutput=off  SatLimitsSource=internal  UpperSaturationLimit=inf  LowerSaturationLimit=-inf  LinearizeAsGain=off  AntiWindupMode=none  Kb=1  LimitIntegrator=off  UpperIntegratorSaturationLimit=inf  LowerIntegratorSaturationLimit=-inf  POutMin=[]  POutMax=[]  IOutMin=[]  IOutMax=[]  DOutMin=[]  DOutMax=[]  NOutMin=[]  NOutMax=[]  SumOutMin=[]  SumOutMax=[]  SaturationOutMin=[]  SaturationOutMax=[]  PParamMin=[]  PParamMax=[]  IParamMin=[]  IParamMax=[]  DParamMin=[]  DParamMax=[]  NParamMin=[]  NParamMax=[]  KbParamMin=[]  KbParamMax=[]  KtParamMin=[]  KtParamMax=[]  KbOutMin=[]  KbOutMax=[]  KtOutMin=[]  KtOutMax=[]  IntegratorOutMin=[]  IntegratorOutMax=[]  FilterOutMin=[]  FilterOutMax=[]  SumI1OutMin=[]  SumI1OutMax=[]  SumI2OutMin=[]  SumI2OutMax=[]  SumI3OutMin=[]  SumI3OutMax=[]  SumI4OutMin=[]  SumI4OutMax=[]  SumDOutMin=[]  SumDOutMax=[]  DifferentiatorOutMin=[]  DifferentiatorOutMax=[]  FilterDiffOutCoefMin=[]  FilterDiffOutCoefMax=[]  ReciprocalOutMin=[]  ReciprocalOutMax=[]  SumDenOutMin=[]  SumDenOutMax=[]  SumNumOutMin=[]  SumNumOutMax=[]  DivideOutMin=[]  DivideOutMax=[]  UdiffTsProdOutMin=[]  UdiffTsProdOutMax=[]  NTsProdOutMin=[]  NTsProdOutMax=[]  UintegralTsProdOutMin=[]  UintegralTsProdOutMax=[]  UngainTsProdOutMin=[]  UngainTsProdOutMax=[]  ClampingZeroOutDataTypeStr=Inherit: Inherit via back propagation  ClampingZeroOutMin=[]  ClampingZeroOutMax=[]  FilterDenConstantOutDataTypeStr=Inherit: Inherit via back propagation  FilterDenConstantOutMin=[]  FilterDenConstantOutMax=[]  PCopyOutDataTypeStr=Inherit: Inherit via back propagation  PCopyOutMin=[]  PCopyOutMax=[]  NCopyOutDataTypeStr=Inherit: Inherit via back propagation  NCopyOutMin=[]  NCopyOutMax=[]  IntegratorContinuousStateAttributes=''  IntegratorStateMustResolveToSignalObject=off  IntegratorRTWStateStorageClass=Auto  FilterContinuousStateAttributes=''  FilterStateMustResolveToSignalObject=off  FilterRTWStateStorageClass=Auto  ParallelPVariant=InternalParameters  IdealPVariant=Disabled  IVariant=InternalParameters  DVariant=InternalParameters  IntegratorVariant=Discrete  SatVariant=Disabled  AWVariant=Passthrough  PCopyVariant=Disabled  TRVariant=Disabled  FdbkBlocksVariant=Forward  IdealPFdbkVariant=Disabled  SatFdbkVariant=Disabled  DerivativeFilterVariant=ForwardEulerFilter  NVariant=InternalParameters  NCopyVariant=Disabled  FilterICVariant=InternalICsFilter  IntegratorICVariant=InternalICs  ExternalResetVariant=Disabled  TRSumVariant=Passthrough  SumFdbkVariant=Disabled  SumVariant=Sum_PID  TsampFilterVariant=InternalTs  TsampNgainVariant=Passthrough  TsampIntegralVariant=Disabled_SignalSpec  ExternalSaturationOutDataTypeStr=Inherit: Same as second input
      settings: LibrarySourceBlock=simulink/Discrete/Discrete PID Controller
  Discrete PID Controller2 : slpidlib/PID Controller  Controller=PID  Form=Parallel  TimeDomain=Discrete-time  UseExternalTs=off  SampleTime=0.05  IntegratorMethod=Forward Euler  FilterMethod=Forward Euler  ControllerParametersSource=internal  P=4.5  I=4.3  UseKiTs=off  D=0  N=100  UseFilter=on  TunerSelectOption=Transfer Function Based (PID Tuner App)  InitialConditionSource=internal  InitialConditionForIntegrator=0  InitialConditionForFilter=0  DifferentiatorICPrevScaledInput=0  ExternalReset=none  TrackingMode=off  Kt=1  LimitOutput=off  SatLimitsSource=internal  UpperSaturationLimit=inf  LowerSaturationLimit=-inf  LinearizeAsGain=off  AntiWindupMode=none  Kb=1  LimitIntegrator=off  UpperIntegratorSaturationLimit=inf  LowerIntegratorSaturationLimit=-inf  POutMin=[]  POutMax=[]  IOutMin=[]  IOutMax=[]  DOutMin=[]  DOutMax=[]  NOutMin=[]  NOutMax=[]  SumOutMin=[]  SumOutMax=[]  SaturationOutMin=[]  SaturationOutMax=[]  PParamMin=[]  PParamMax=[]  IParamMin=[]  IParamMax=[]  DParamMin=[]  DParamMax=[]  NParamMin=[]  NParamMax=[]  KbParamMin=[]  KbParamMax=[]  KtParamMin=[]  KtParamMax=[]  KbOutMin=[]  KbOutMax=[]  KtOutMin=[]  KtOutMax=[]  IntegratorOutMin=[]  IntegratorOutMax=[]  FilterOutMin=[]  FilterOutMax=[]  SumI1OutMin=[]  SumI1OutMax=[]  SumI2OutMin=[]  SumI2OutMax=[]  SumI3OutMin=[]  SumI3OutMax=[]  SumI4OutMin=[]  SumI4OutMax=[]  SumDOutMin=[]  SumDOutMax=[]  DifferentiatorOutMin=[]  DifferentiatorOutMax=[]  FilterDiffOutCoefMin=[]  FilterDiffOutCoefMax=[]  ReciprocalOutMin=[]  ReciprocalOutMax=[]  SumDenOutMin=[]  SumDenOutMax=[]  SumNumOutMin=[]  SumNumOutMax=[]  DivideOutMin=[]  DivideOutMax=[]  UdiffTsProdOutMin=[]  UdiffTsProdOutMax=[]  NTsProdOutMin=[]  NTsProdOutMax=[]  UintegralTsProdOutMin=[]  UintegralTsProdOutMax=[]  UngainTsProdOutMin=[]  UngainTsProdOutMax=[]  ClampingZeroOutDataTypeStr=Inherit: Inherit via back propagation  ClampingZeroOutMin=[]  ClampingZeroOutMax=[]  FilterDenConstantOutDataTypeStr=Inherit: Inherit via back propagation  FilterDenConstantOutMin=[]  FilterDenConstantOutMax=[]  PCopyOutDataTypeStr=Inherit: Inherit via back propagation  PCopyOutMin=[]  PCopyOutMax=[]  NCopyOutDataTypeStr=Inherit: Inherit via back propagation  NCopyOutMin=[]  NCopyOutMax=[]  IntegratorContinuousStateAttributes=''  IntegratorStateMustResolveToSignalObject=off  IntegratorRTWStateStorageClass=Auto  FilterContinuousStateAttributes=''  FilterStateMustResolveToSignalObject=off  FilterRTWStateStorageClass=Auto  ParallelPVariant=InternalParameters  IdealPVariant=Disabled  IVariant=InternalParameters  DVariant=InternalParameters  IntegratorVariant=Discrete  SatVariant=Disabled  AWVariant=Passthrough  PCopyVariant=Disabled  TRVariant=Disabled  FdbkBlocksVariant=Forward  IdealPFdbkVariant=Disabled  SatFdbkVariant=Disabled  DerivativeFilterVariant=ForwardEulerFilter  NVariant=InternalParameters  NCopyVariant=Disabled  FilterICVariant=InternalICsFilter  IntegratorICVariant=InternalICs  ExternalResetVariant=Disabled  TRSumVariant=Passthrough  SumFdbkVariant=Disabled  SumVariant=Sum_PID  TsampFilterVariant=InternalTs  TsampNgainVariant=Passthrough  TsampIntegralVariant=Disabled_SignalSpec  ExternalSaturationOutDataTypeStr=Inherit: Same as second input
      settings: LibrarySourceBlock=simulink/Discrete/Discrete PID Controller
  Gain : Gain
  Gain1 : Gain
  Mux1 : Mux  Inputs=3
  Scope : Scope
  Scope1 : Scope
  Scope2 : Scope
  Zero-Order Hold3 : ZeroOrderHold  SampleTime=0.05
  Zero-Order Hold4 : ZeroOrderHold  SampleTime=0.05
  Zero-Order Hold5 : ZeroOrderHold  SampleTime=0.05
  vx* : Outport
  vy* : Outport  Port=2
  vz* : Outport  Port=3
  sampled_error : Outport  Port=4
  wires:
  Discrete PID Controller2/1 -> vz*/1
  Discrete PID Controller1/1 -> vy*/1
  Discrete PID Controller/1 -> vx*/1
  Add1/1 -> Add5/2
  Constant/1 -> Add3/2
  Add/1 -> Add3/1  "ground truth error_x"
  z_ee*/1 -> Add1/2
  y_ee*/1 -> Add2/2
  Constant2/1 -> Add5/1
  Zero-Order Hold5/1 -> Discrete PID Controller2/1, Mux1/3
  Add4/1 -> Gain1/1
  x_ee*/1 -> Add/2
  x_ee/1 -> Add/1
  Add5/1 -> Zero-Order Hold5/1, Scope2/1
  Zero-Order Hold3/1 -> Discrete PID Controller/1, Scope/1, Mux1/1  "sampled slow error_x"
  y_ee/1 -> Add2/1
  Add2/1 -> Add4/1
  Constant1/1 -> Add4/2
  Zero-Order Hold4/1 -> Discrete PID Controller1/1, Scope1/1, Mux1/2
  z_ee/1 -> Add1/1
  Add3/1 -> Gain/1  "ground truth error_x"
  Mux1/1 -> sampled_error/1
  Gain/1 -> Zero-Order Hold3/1
  Gain1/1 -> Zero-Order Hold4/1

== system ur5_simulink_ros2_pbvs_all_methods_2023b/Subsystem ==
  u : Inport
  Enable : EnablePort
  Bus Creator2 : BusCreator  Inputs=3
  MATLAB Function : MATLAB Function  TreatAsAtomicUnit=on
  X_in : Outport
  wires:
  MATLAB Function/2(y) -> Bus Creator2/2
  MATLAB Function/1(x) -> Bus Creator2/1
  MATLAB Function/3(z) -> Bus Creator2/3
  u/1 -> MATLAB Function/1(u)
  Bus Creator2/1 -> X_in/1

== system ur5_simulink_ros2_pbvs_all_methods_2023b/Subsystem3 ==
  u : Inport
  Enable : EnablePort
  MATLAB Function : MATLAB Function  TreatAsAtomicUnit=on
  joint1_pos : Outport
  joint2_pos : Outport  Port=2
  joint3_pos : Outport  Port=3
  joint4_pos : Outport  Port=4
  joint5_pos : Outport  Port=5
  joint6_pos : Outport  Port=6
  wires:
  u/1 -> MATLAB Function/1(u)
  MATLAB Function/1(joint1_pos) -> joint1_pos/1
  MATLAB Function/2(joint2_pos) -> joint2_pos/1
  MATLAB Function/3(joint3_pos) -> joint3_pos/1
  MATLAB Function/4(joint4_pos) -> joint4_pos/1
  MATLAB Function/5(joint5_pos) -> joint5_pos/1
  MATLAB Function/6(joint6_pos) -> joint6_pos/1

== system ur5_simulink_ros2_pbvs_all_methods_2023b/Subsystem4 ==
  motor_state : Inport
  Blank Message : ros2lib/Blank Message  messageClass=Message  entityType=std_msgs/Int64  messageType=std_msgs/Int64  SampleTime=inf
  Bus Assignment1 : BusAssignment  AssignedSignals=data
  y : Outport
  wires:
  Blank Message/1 -> Bus Assignment1/1
  Bus Assignment1/1 -> y/1
  motor_state/1 -> Bus Assignment1/2

== system ur5_simulink_ros2_pbvs_all_methods_2023b/Subsystem5 ==
  R_current : Inport
  Discrete Pulse Generator : DiscretePulseGenerator  SampleTime=0.005
  attitude_pi_ctrl : Subsystem
  u : Outport
  wires:
  Discrete Pulse Generator/1 -> attitude_pi_ctrl/Trigger
  R_current/1 -> attitude_pi_ctrl/1(R_current)
  attitude_pi_ctrl/1(u) -> u/1

== system ur5_simulink_ros2_pbvs_all_methods_2023b/joint vel to ros3 ==
  u : Inport
  flag : Inport  Port=2
  Blank Message1 : ros2lib/Blank Message  messageClass=Message  entityType=std_msgs/Float64MultiArray  messageType=std_msgs/Float64MultiArray  SampleTime=inf
      settings: LibrarySourceBlock=roslib/ROS 2/Blank Message
  Bus Assignment1 : BusAssignment  AssignedSignals=data,data_SL_Info.CurrentLength,data_SL_Info.ReceivedLength
  Constant : Constant  Value=128  OutDataTypeStr=uint32
  Constant{1,3..7} (6 alike) : Constant  Value=0
  Constant2 : Constant  Value=128  OutDataTypeStr=uint32
  to ros2 : MATLAB Function  TreatAsAtomicUnit=on
  Out1 : Outport
  wires:
  u/1 -> to ros2/1(u)
  Constant2/1 -> Bus Assignment1/4
  Constant/1 -> Bus Assignment1/3
  Blank Message1/1 -> Bus Assignment1/1
  Bus Assignment1/1 -> Out1/1
  Constant5/1 -> to ros2/3(joint1)
  Constant1/1 -> to ros2/4(joint2)
  Constant3/1 -> to ros2/5(joint3)
  Constant4/1 -> to ros2/6(joint4)
  Constant6/1 -> to ros2/7(joint5)
  Constant7/1 -> to ros2/8(joint6)
  flag/1 -> to ros2/2(flag)
  to ros2/1(y) -> Bus Assignment1/2

== system ur5_simulink_ros2_pbvs_all_methods_2023b/AIC/Subsystem1 ==
  y1_real_slow : Inport
  y2_derivative_sampling : Inport  Port=2
  AIC_muti_sensor_module : Subsystem
  Discrete Pulse Generator : DiscretePulseGenerator  Period=10  SampleTime=0.005
  mu : Outport
  mu_p : Outport  Port=2
  u : Outport  Port=3
  wires:
  AIC_muti_sensor_module/1(u) -> u/1  "u"
  y1_real_slow/1 -> AIC_muti_sensor_module/1(y1_real_slow)
  y2_derivative_sampling/1 -> AIC_muti_sensor_module/2(y2_derivative_sampling)
  Discrete Pulse Generator/1 -> AIC_muti_sensor_module/Trigger
  AIC_muti_sensor_module/3(mu_p) -> mu_p/1
  AIC_muti_sensor_module/2(mu) -> mu/1

== system ur5_simulink_ros2_pbvs_all_methods_2023b/AIC/Subsystem2 ==
  y1_real_slow : Inport
  y2_derivative_sampling : Inport  Port=2
  AIC_muti_sensor_module : Subsystem
  Discrete Pulse Generator : DiscretePulseGenerator  Period=10  SampleTime=0.005
  mu : Outport
  mu_p : Outport  Port=2
  u : Outport  Port=3
  wires:
  AIC_muti_sensor_module/1(u) -> u/1  "u"
  y1_real_slow/1 -> AIC_muti_sensor_module/1(y1_real_slow)
  y2_derivative_sampling/1 -> AIC_muti_sensor_module/2(y2_derivative_sampling)
  Discrete Pulse Generator/1 -> AIC_muti_sensor_module/Trigger
  AIC_muti_sensor_module/3(mu_p) -> mu_p/1
  AIC_muti_sensor_module/2(mu) -> mu/1

== system ur5_simulink_ros2_pbvs_all_methods_2023b/AIC/Subsystem3 ==
  y1_real_slow : Inport
  y2_derivative_sampling : Inport  Port=2
  AIC_muti_sensor_module : Subsystem
  Discrete Pulse Generator : DiscretePulseGenerator  Period=10  SampleTime=0.005
  mu : Outport
  mu_p : Outport  Port=2
  u : Outport  Port=3
  wires:
  AIC_muti_sensor_module/1(u) -> u/1  "u"
  y1_real_slow/1 -> AIC_muti_sensor_module/1(y1_real_slow)
  y2_derivative_sampling/1 -> AIC_muti_sensor_module/2(y2_derivative_sampling)
  Discrete Pulse Generator/1 -> AIC_muti_sensor_module/Trigger
  AIC_muti_sensor_module/3(mu_p) -> mu_p/1
  AIC_muti_sensor_module/2(mu) -> mu/1

== system ur5_simulink_ros2_pbvs_all_methods_2023b/F-PID/Subsystem1 ==
  y1_real_slow : Inport
  Demux : Demux  Outputs=2
  Discrete Pulse Generator1 : DiscretePulseGenerator  SampleTime=0.005
  F-PID : Subsystem
  hat_y1_100hz : Outport
  u : Outport  Port=2
  wires:
  y1_real_slow/1 -> F-PID/1(y1_real_slow)
  Discrete Pulse Generator1/1 -> F-PID/Trigger
  F-PID/2(u) -> u/1
  F-PID/1(hat_x) -> Demux/1
  Demux/1 -> hat_y1_100hz/1

== system ur5_simulink_ros2_pbvs_all_methods_2023b/F-PID/Subsystem2 ==
  y1_real_slow : Inport
  Demux : Demux  Outputs=2
  Discrete Pulse Generator1 : DiscretePulseGenerator  SampleTime=0.005
  F-PID : Subsystem
  hat_y1_100hz : Outport
  u : Outport  Port=2
  wires:
  y1_real_slow/1 -> F-PID/1(y1_real_slow)
  Discrete Pulse Generator1/1 -> F-PID/Trigger
  F-PID/2(u) -> u/1
  F-PID/1(hat_x) -> Demux/1
  Demux/1 -> hat_y1_100hz/1

== system ur5_simulink_ros2_pbvs_all_methods_2023b/F-PID/Subsystem3 ==
  y1_real_slow : Inport
  Demux : Demux  Outputs=2
  Discrete Pulse Generator1 : DiscretePulseGenerator  SampleTime=0.005
  F-PID : Subsystem
  hat_y1_100hz : Outport
  u : Outport  Port=2
  wires:
  y1_real_slow/1 -> F-PID/1(y1_real_slow)
  Discrete Pulse Generator1/1 -> F-PID/Trigger
  F-PID/2(u) -> u/1
  F-PID/1(hat_x) -> Demux/1
  Demux/1 -> hat_y1_100hz/1

== system ur5_simulink_ros2_pbvs_all_methods_2023b/MPC-DOB/mpc ==
  ex : Inport
  Constant : Constant  Value=0
  Delay1 : Delay  DelayLength=1  SampleTime=0.05
  MPC Controller : mpclib/MPC Controller  SCDEnableBlockLinearizationSpecification=on  mpcobj=mpcobj  is_multiple=0  enable_value=0  return_u0=off  updateMPCinCallerWorkspace=on  md_inport=on  mv_inport=off  uref_inport=off  return_cost=off  return_mvseq=off  return_qpstatus=off  return_xseq=off  return_state=off  return_ovseq=off  state_inport=off  umin_inport=off  umax_inport=off  ymin_inport=off  ymax_inport=off  cc_inport=off  ywt_inport=off  uwt_inport=off  duwt_inport=off  rhoeps_inport=off  pm_inport=off  MaximumP=10  HorizonChoice=FixedHorizon  n_ts=0.05  n_p=20  n_mv=1  n_md=1  n_ud=0  n_mo=1  n_uo=0  BlockDataType=double  SampleTimeInherited=on  switch_inport=off
  Pulse Generator : DiscretePulseGenerator  Period=5  SampleTime=0.01
  Subsystem : Subsystem
  mv : Outport
  wires:
  MPC Controller/1 -> mv/1, Subsystem/2(u)
  ex/1 -> MPC Controller/1, Subsystem/1(ex)
  Subsystem/1(dhat) -> Delay1/1
  Constant/1 -> MPC Controller/2
  Delay1/1 -> MPC Controller/3
  Pulse Generator/1 -> Subsystem/Trigger

== system ur5_simulink_ros2_pbvs_all_methods_2023b/MPC-DOB/mpc1 ==
  ex : Inport
  Constant : Constant  Value=0
  Delay1 : Delay  DelayLength=1  SampleTime=0.05
  MPC Controller : mpclib/MPC Controller  SCDEnableBlockLinearizationSpecification=on  mpcobj=mpcobj  is_multiple=0  enable_value=0  return_u0=off  updateMPCinCallerWorkspace=on  md_inport=on  mv_inport=off  uref_inport=off  return_cost=off  return_mvseq=off  return_qpstatus=off  return_xseq=off  return_state=off  return_ovseq=off  state_inport=off  umin_inport=off  umax_inport=off  ymin_inport=off  ymax_inport=off  cc_inport=off  ywt_inport=off  uwt_inport=off  duwt_inport=off  rhoeps_inport=off  pm_inport=off  MaximumP=10  HorizonChoice=FixedHorizon  n_ts=0.05  n_p=20  n_mv=1  n_md=1  n_ud=0  n_mo=1  n_uo=0  BlockDataType=double  SampleTimeInherited=on  switch_inport=off
  Pulse Generator : DiscretePulseGenerator  Period=5  SampleTime=0.01
  Subsystem : Subsystem
  mv : Outport
  wires:
  MPC Controller/1 -> mv/1, Subsystem/2(u)
  ex/1 -> MPC Controller/1, Subsystem/1(ex)
  Subsystem/1(dhat) -> Delay1/1
  Constant/1 -> MPC Controller/2
  Delay1/1 -> MPC Controller/3
  Pulse Generator/1 -> Subsystem/Trigger

== system ur5_simulink_ros2_pbvs_all_methods_2023b/MPC-DOB/mpc2 ==
  ex : Inport
  Constant : Constant  Value=0
  Delay1 : Delay  DelayLength=1  SampleTime=0.05
  MPC Controller : mpclib/MPC Controller  SCDEnableBlockLinearizationSpecification=on  mpcobj=mpcobj  is_multiple=0  enable_value=0  return_u0=off  updateMPCinCallerWorkspace=on  md_inport=on  mv_inport=off  uref_inport=off  return_cost=off  return_mvseq=off  return_qpstatus=off  return_xseq=off  return_state=off  return_ovseq=off  state_inport=off  umin_inport=off  umax_inport=off  ymin_inport=off  ymax_inport=off  cc_inport=off  ywt_inport=off  uwt_inport=off  duwt_inport=off  rhoeps_inport=off  pm_inport=off  MaximumP=10  HorizonChoice=FixedHorizon  n_ts=0.05  n_p=20  n_mv=1  n_md=1  n_ud=0  n_mo=1  n_uo=0  BlockDataType=double  SampleTimeInherited=on  switch_inport=off
  Pulse Generator : DiscretePulseGenerator  Period=5  SampleTime=0.01
  Subsystem : Subsystem
  mv : Outport
  wires:
  MPC Controller/1 -> mv/1, Subsystem/2(u)
  ex/1 -> MPC Controller/1, Subsystem/1(ex)
  Subsystem/1(dhat) -> Delay1/1
  Constant/1 -> MPC Controller/2
  Delay1/1 -> MPC Controller/3
  Pulse Generator/1 -> Subsystem/Trigger

== system ur5_simulink_ros2_pbvs_all_methods_2023b/RAID-AgIVS/Subsystem1 ==
  y1_real_slow : Inport
  y2_derivative_sampling : Inport  Port=2
  APO+AIC : Subsystem
  Discrete Pulse Generator1 : DiscretePulseGenerator  SampleTime=0.005
  Selector : Selector  InputPortWidth=2  IndexOptions=Index vector (dialog)  Indices=[1]  OutputSizes=1
  Selector1 : Selector  InputPortWidth=2  IndexOptions=Index vector (dialog)  Indices=[2]  OutputSizes=1
  hat_y1_100hz : Outport
  hat_y2_100hz : Outport  Port=2
  u : Outport  Port=3
  wires:
  y1_real_slow/1 -> APO+AIC/1(y1_real_slow)
  y2_derivative_sampling/1 -> APO+AIC/2(y2_real_slow)
  Selector1/1 -> hat_y2_100hz/1
  Discrete Pulse Generator1/1 -> APO+AIC/Trigger
  APO+AIC/1(hat_x) -> Selector/1, Selector1/1
  Selector/1 -> hat_y1_100hz/1
  APO+AIC/2(u) -> u/1

== system ur5_simulink_ros2_pbvs_all_methods_2023b/RAID-AgIVS/Subsystem2 ==
  y1_real_slow : Inport
  y2_derivative_sampling : Inport  Port=2
  APO+AIC : Subsystem
  Discrete Pulse Generator1 : DiscretePulseGenerator  SampleTime=0.005
  Selector : Selector  InputPortWidth=2  IndexOptions=Index vector (dialog)  Indices=[1]  OutputSizes=1
  Selector1 : Selector  InputPortWidth=2  IndexOptions=Index vector (dialog)  Indices=[2]  OutputSizes=1
  hat_y1_100hz : Outport
  hat_y2_100hz : Outport  Port=2
  u : Outport  Port=3
  wires:
  y1_real_slow/1 -> APO+AIC/1(y1_real_slow)
  y2_derivative_sampling/1 -> APO+AIC/2(y2_real_slow)
  Selector1/1 -> hat_y2_100hz/1
  Discrete Pulse Generator1/1 -> APO+AIC/Trigger
  APO+AIC/1(hat_x) -> Selector/1, Selector1/1
  Selector/1 -> hat_y1_100hz/1
  APO+AIC/2(u) -> u/1

== system ur5_simulink_ros2_pbvs_all_methods_2023b/RAID-AgIVS/Subsystem3 ==
  y1_real_slow : Inport
  y2_derivative_sampling : Inport  Port=2
  APO+AIC : Subsystem
  Discrete Pulse Generator1 : DiscretePulseGenerator  SampleTime=0.005
  Selector : Selector  InputPortWidth=2  IndexOptions=Index vector (dialog)  Indices=[1]  OutputSizes=1
  Selector1 : Selector  InputPortWidth=2  IndexOptions=Index vector (dialog)  Indices=[2]  OutputSizes=1
  hat_y1_100hz : Outport
  hat_y2_100hz : Outport  Port=2
  u : Outport  Port=3
  wires:
  y1_real_slow/1 -> APO+AIC/1(y1_real_slow)
  y2_derivative_sampling/1 -> APO+AIC/2(y2_real_slow)
  Selector1/1 -> hat_y2_100hz/1
  Discrete Pulse Generator1/1 -> APO+AIC/Trigger
  APO+AIC/1(hat_x) -> Selector/1, Selector1/1
  Selector/1 -> hat_y1_100hz/1
  APO+AIC/2(u) -> u/1

== system ur5_simulink_ros2_pbvs_all_methods_2023b/Subsystem5/attitude_pi_ctrl ==
  R_current : Inport
  Trigger : TriggerPort  VariantControl=(inherit)  PortDimensions=1
  MATLAB Function : MATLAB Function  TreatAsAtomicUnit=on
  u : Outport
  wires:
  R_current/1 -> MATLAB Function/1(R_current)
  MATLAB Function/1(u) -> u/1

== system ur5_simulink_ros2_pbvs_all_methods_2023b/AIC/Subsystem1/AIC_muti_sensor_module ==
  y1_real_slow : Inport
  y2_derivative_sampling : Inport  Port=2
  10ms : TriggerPort  VariantControl=(inherit)  InitialTriggerSignalState=zero  PortDimensions=1
  Cast To Double : DataTypeConversion  OutDataTypeStr=double  SaturateOnIntegerOverflow=off  RndMeth=Floor
  Cast To Double1 : DataTypeConversion  OutDataTypeStr=double  SaturateOnIntegerOverflow=off  RndMeth=Floor
  Cast To Double2 : DataTypeConversion  OutDataTypeStr=double  SaturateOnIntegerOverflow=off  RndMeth=Floor
  Discrete Derivative : simulink/Discrete/Discrete Derivative  gainval=1.0  ICPrevScaledInput=0.0  OutMin=[]  OutMax=[]  OutDataType=fixdt(1, 16)  OutScaling=2^-10  DoSatur=off
  MATLAB Function : MATLAB Function  TreatAsAtomicUnit=on
  Memory : Memory  InheritSampleTime=on
  Memory1 : Memory  InheritSampleTime=on
  Memory2 : Memory  InheritSampleTime=on
  u : Outport
  mu : Outport  Port=2
  mu_p : Outport  Port=3
  wires:
  Memory2/1 -> Cast To Double/1
  Memory/1 -> Cast To Double2/1
  y1_real_slow/1 -> MATLAB Function/1(y1_real_slow)
  MATLAB Function/1(u) -> Memory/1, u/1
  MATLAB Function/3(mu_p) -> mu_p/1, Memory2/1
  Memory1/1 -> Cast To Double1/1
  MATLAB Function/2(mu) -> mu/1, Memory1/1
  Cast To Double/1 -> MATLAB Function/4(mu_p_last)
  Cast To Double1/1 -> MATLAB Function/3(mu_last)
  Cast To Double2/1 -> MATLAB Function/5(u_last)
  y2_derivative_sampling/1 -> MATLAB Function/2(y2_derivative_sampling)

== system ur5_simulink_ros2_pbvs_all_methods_2023b/AIC/Subsystem2/AIC_muti_sensor_module ==
  y1_real_slow : Inport
  y2_derivative_sampling : Inport  Port=2
  10ms : TriggerPort  VariantControl=(inherit)  InitialTriggerSignalState=zero  PortDimensions=1
  Cast To Double : DataTypeConversion  OutDataTypeStr=double  SaturateOnIntegerOverflow=off  RndMeth=Floor
  Cast To Double1 : DataTypeConversion  OutDataTypeStr=double  SaturateOnIntegerOverflow=off  RndMeth=Floor
  Cast To Double2 : DataTypeConversion  OutDataTypeStr=double  SaturateOnIntegerOverflow=off  RndMeth=Floor
  Discrete Derivative : simulink/Discrete/Discrete Derivative  gainval=1.0  ICPrevScaledInput=0.0  OutMin=[]  OutMax=[]  OutDataType=fixdt(1, 16)  OutScaling=2^-10  DoSatur=off
  MATLAB Function : MATLAB Function  TreatAsAtomicUnit=on
  Memory : Memory  InheritSampleTime=on
  Memory1 : Memory  InheritSampleTime=on
  Memory2 : Memory  InheritSampleTime=on
  u : Outport
  mu : Outport  Port=2
  mu_p : Outport  Port=3
  wires:
  Memory2/1 -> Cast To Double/1
  Memory/1 -> Cast To Double2/1
  y1_real_slow/1 -> MATLAB Function/1(y1_real_slow)
  MATLAB Function/1(u) -> Memory/1, u/1
  MATLAB Function/3(mu_p) -> mu_p/1, Memory2/1
  Memory1/1 -> Cast To Double1/1
  MATLAB Function/2(mu) -> mu/1, Memory1/1
  Cast To Double/1 -> MATLAB Function/4(mu_p_last)
  Cast To Double1/1 -> MATLAB Function/3(mu_last)
  Cast To Double2/1 -> MATLAB Function/5(u_last)
  y2_derivative_sampling/1 -> MATLAB Function/2(y2_derivative_sampling)

== system ur5_simulink_ros2_pbvs_all_methods_2023b/AIC/Subsystem3/AIC_muti_sensor_module ==
  y1_real_slow : Inport
  y2_derivative_sampling : Inport  Port=2
  10ms : TriggerPort  VariantControl=(inherit)  InitialTriggerSignalState=zero  PortDimensions=1
  Cast To Double : DataTypeConversion  OutDataTypeStr=double  SaturateOnIntegerOverflow=off  RndMeth=Floor
  Cast To Double1 : DataTypeConversion  OutDataTypeStr=double  SaturateOnIntegerOverflow=off  RndMeth=Floor
  Cast To Double2 : DataTypeConversion  OutDataTypeStr=double  SaturateOnIntegerOverflow=off  RndMeth=Floor
  Discrete Derivative : simulink/Discrete/Discrete Derivative  gainval=1.0  ICPrevScaledInput=0.0  OutMin=[]  OutMax=[]  OutDataType=fixdt(1, 16)  OutScaling=2^-10  DoSatur=off
  MATLAB Function : MATLAB Function  TreatAsAtomicUnit=on
  Memory : Memory  InheritSampleTime=on
  Memory1 : Memory  InheritSampleTime=on
  Memory2 : Memory  InheritSampleTime=on
  u : Outport
  mu : Outport  Port=2
  mu_p : Outport  Port=3
  wires:
  Memory2/1 -> Cast To Double/1
  Memory/1 -> Cast To Double2/1
  y1_real_slow/1 -> MATLAB Function/1(y1_real_slow)
  MATLAB Function/1(u) -> Memory/1, u/1
  MATLAB Function/3(mu_p) -> mu_p/1, Memory2/1
  Memory1/1 -> Cast To Double1/1
  MATLAB Function/2(mu) -> mu/1, Memory1/1
  Cast To Double/1 -> MATLAB Function/4(mu_p_last)
  Cast To Double1/1 -> MATLAB Function/3(mu_last)
  Cast To Double2/1 -> MATLAB Function/5(u_last)
  y2_derivative_sampling/1 -> MATLAB Function/2(y2_derivative_sampling)
